simulink model "mode"  (R2021b)
settings: Solver=ode23s  StartTime=0.0  StopTime=50  RelTol=1e-3
model workspace (MAT data in the model file):
  firstWarning = 1
  originalScenarioChecksum = '114339432DE22364D47BB28FC96DC10C'
undefined symbols (not defined in the file or in its folder): Acceleration, ActorID, AngularVelocity, curvature, DefaultGear, DEND_B, DEND_S, DEND_T, direction, driving, gradbp, LF, LR, matlabshared, MAX_BRAKE, MAX_STEER, MAX_TORQUE, MCAR, MIN_BRAKE, MIN_STEER, MIN_TORQUE, NUMD_B, NUMD_S, NUMD_T, Pitch, point_intersection, Position, psi_o, R, Roll, RRdamp, scenario, sigbuilder_block, STEER_RATIO, stopSign_ID, Tdead, thetaRefs, TL_ID, TrackWidth, Ts, ts, Vdead, Velocity, X_o, xRef2s, Y_o, Yaw, yRef2s
libraries: drivingscenarioandsensors x4, drivingvehiclecontroller x2, simulink x2, simulink_extras x1, autolibshared x1, vehdynlibviscommon x1, vehdynlibsteering x1
(part 2 of 2)

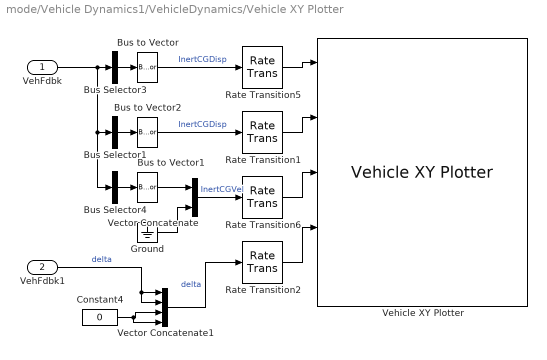
== system mode/Vehicle Dynamics1/VehicleDynamics/Vehicle XY Plotter ==
  VehFdbk : Inport
  VehFdbk1 : Inport  Port=2
  Bus Selector1 : BusSelector  OutputSignals=InertFrm.Cg.Ang.phi,InertFrm.Cg.Ang.theta,InertFrm.Cg.Ang.psi  OutputAsBus=on
  Bus Selector3 : BusSelector  OutputSignals=InertFrm.Geom.Disp.X,InertFrm.Geom.Disp.Y,InertFrm.Geom.Disp.Z  OutputAsBus=on
  Bus Selector4 : BusSelector  OutputSignals=InertFrm.Cg.Vel.Xdot,InertFrm.Cg.Vel.Ydot  OutputAsBus=on
  Bus to Vector : BusToVector
  Bus to Vector1 : BusToVector
  Bus to Vector2 : BusToVector
  Constant4 : Constant  Value=0
  Ground : Ground
  Rate Transition{1..2,5..6} (4 alike) : RateTransition  OutPortSampleTime=pltDT
  Vector Concatenate : Concatenate
  Vector Concatenate1 : Concatenate  NumInputs=4
  Vehicle XY Plotter : vehdynlibviscommon/Vehicle XY Plotter  w=w  a=a  b=b  figBorder=2000  bufferSize=bufferSize  extStats=off  extTireF=off
      settings: SourceProductName=The database C:\Users\jrodgers\AppData\Roaming\MathWorks\MATLAB\R2018b\slblocks_master.db is locked, or a table in the database is locked. (database is locked)
  wires:
  Bus to Vector2/1 -> Rate Transition1/1  "InertCGDisp"
  Rate Transition5/1 -> Vehicle XY Plotter/1
  Bus Selector4/1 -> Bus to Vector1/1
  Rate Transition1/1 -> Vehicle XY Plotter/2
  Rate Transition6/1 -> Vehicle XY Plotter/3
  Vector Concatenate/1 -> Rate Transition6/1  "InertCGVel"
  Bus Selector1/1 -> Bus to Vector2/1
  Bus to Vector/1 -> Rate Transition5/1  "InertCGDisp"
  Bus Selector3/1 -> Bus to Vector/1
  Bus to Vector1/1 -> Vector Concatenate/1
  Ground/1 -> Vector Concatenate/2
  VehFdbk/1 -> Bus Selector1/1, Bus Selector4/1, Bus Selector3/1
  Rate Transition2/1 -> Vehicle XY Plotter/4
  Constant4/1 -> Vector Concatenate1/4, Vector Concatenate1/3
  VehFdbk1/1 -> Vector Concatenate1/2, Vector Concatenate1/1  "delta"
  Vector Concatenate1/1 -> Rate Transition2/1  "delta"

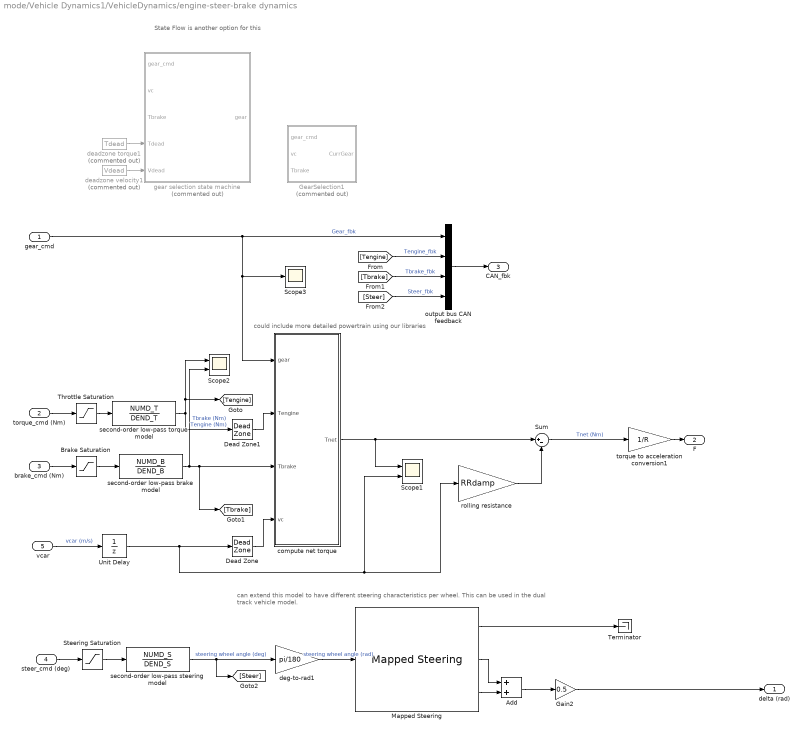
== system mode/Vehicle Dynamics1/VehicleDynamics/engine-steer-brake dynamics ==
  note: State Flow is another option for this
  note: could include more detailed powertrain using our libraries
  note: can extend this model to have different steering characteristics per wheel. This can be used in the dual track vehicle model.
  gear_cmd : Inport
  torque_cmd (Nm) : Inport  Port=2
  brake_cmd (Nm) : Inport  Port=3
  steer_cmd (deg) : Inport  Port=4
  vcar : Inport  Port=5
  Add : Sum
  Brake Saturation : Saturate  UpperLimit=MAX_BRAKE  LowerLimit=MIN_BRAKE
  Dead Zone : DeadZone  LowerValue=-Vdead  UpperValue=Vdead  SaturateOnIntegerOverflow=on
  Dead Zone1 : DeadZone  LowerValue=-Tdead  UpperValue=Tdead  SaturateOnIntegerOverflow=on
  Gain2 : Gain  Gain=0.5
  GearSelection1 : Stateflow chart  Commented=on  TreatAsAtomicUnit=on  SystemSampleTime=ts
      settings: PortSchema="{\"entries\":[{\"content\":{\"sides\":[{\"content\":{\"connectorIds\":[\"In3\",\"In2\",\"In1\"]},\"type\":\"ConnectorPlacement.EquallySpacedRectSide\",\"uuid\":\"465e5722-891f-481b-b3b6-2b8339e8e743\"},{\"content\":{\"connectorIds\":[\"Out1\"],\"side\":\"RIGHT\"},\"type\":\"ConnectorPlacement.EquallySpacedRectSide\",\"uuid\":\"28ef13cd-41d9-4e2e-8cd9-9157abf573a9\"},{\"content\":{\"connectorIds\":[],\"side\":\"TOP\"},\"type\":\"ConnectorPlacement.EquallySpacedRectSide\",\"uuid\":\"44f19923-60ae-466f-ad2a-756f1033b52e\"},{\"content\":{\"connectorIds\":[],\"side\":\"HIDDEN\"},\"type\":\"ConnectorPlacement.EquallySpacedRectSide\",\"uuid\":\"d5a146f0-4328-42be-94e3-09f51634e7da\"}]},\"type\":\"ConnectorPlacement.EquallySpacedConnector\",\"uuid\":\"14e271af-3da2-4f7d-9688-fcc3c9792006\"}],\"packageUris\":[\"http://schema.mathworks.com/mf0/Connector/R2020b\"],\"version\":\"1.0\"}"
  Mapped Steering : vehdynlibsteering/Mapped Steering  SpdDpd=off  StrgAngBpts=[-1.5*pi 1.5*pi]  WhlLftTbl=[-1.5*pi 1.5*pi]*STEER_RATIO  WhlRghtTbl=[-1.5*pi 1.5*pi]*STEER_RATIO  VehSpdBpts=[-1 1]  SpdFctTbl=[1 1]  aMode=2
      settings: SourceProductBaseCode=VE
  Scope1 : Scope  NumInputPorts=2
  Scope2 : Scope  NumInputPorts=2
  Scope3 : Scope
  Steering Saturation : Saturate  UpperLimit=MAX_STEER  LowerLimit=MIN_STEER
  Sum : Sum  Inputs=|+-
  Terminator : Terminator
  Throttle Saturation : Saturate  UpperLimit=MAX_TORQUE  LowerLimit=MIN_TORQUE
  Unit Delay : UnitDelay  SampleTime=-1  HasFrameUpgradeWarning=on
  compute net torque : MATLAB Function  TreatAsAtomicUnit=on  SystemSampleTime=ts
  deadzone torque1 : Constant  Commented=on  Value=Tdead  SampleTime=ts
  deadzone velocity1 : Constant  Commented=on  Value=Vdead  SampleTime=ts
  deg-to-rad1 : Gain  Gain=pi/180
  gear selection state machine : MATLAB Function  Commented=on  TreatAsAtomicUnit=on  SystemSampleTime=ts
  output bus CAN feedback : BusCreator  Inputs=4
  rolling resistance : Gain  Gain=RRdamp
  second-order low-pass brake model : DiscreteTransferFcn  Numerator=NUMD_B  Denominator=DEND_B  SampleTime=ts
  second-order low-pass steering model : DiscreteTransferFcn  Numerator=NUMD_S  Denominator=DEND_S  SampleTime=ts
  second-order low-pass torque model : DiscreteTransferFcn  Numerator=NUMD_T  Denominator=DEND_T  SampleTime=ts
  torque to acceleration conversion1 : Gain  Gain=1/R
  delta (rad) : Outport  VectorParamsAs1DForOutWhenUnconnected=off
  F : Outport  Port=2  VectorParamsAs1DForOutWhenUnconnected=off
  CAN_fbk : Outport  Port=3  VectorParamsAs1DForOutWhenUnconnected=off
  wires:
  steer_cmd (deg)/1 -> Steering Saturation/1
  torque_cmd (Nm)/1 -> Throttle Saturation/1
  brake_cmd (Nm)/1 -> Brake Saturation/1
  second-order low-pass steering model/1 -> deg-to-rad1/1, [Steer]  "steering wheel angle (deg)"
  Throttle Saturation/1 -> second-order low-pass torque model/1
  Brake Saturation/1 -> second-order low-pass brake model/1
  Steering Saturation/1 -> second-order low-pass steering model/1
  vcar/1 -> Unit Delay/1  "vcar (m/s)"
  second-order low-pass brake model/1 -> [Tbrake], compute net torque/3(Tbrake), Scope2/2  "Tbrake (Nm)"
  second-order low-pass torque model/1 -> Dead Zone1/1, [Tengine], Scope2/1  "Tengine (Nm)"
  compute net torque/1(Tnet) -> Scope1/1, Sum/1
  rolling resistance/1 -> Sum/2
  deadzone velocity1/1 -> gear selection state machine/5(Vdead)
  deadzone torque1/1 -> gear selection state machine/4(Tdead)
  gear_cmd/1 -> output bus CAN feedback/1, Scope3/1, compute net torque/1(gear)  "Gear_fbk"
  output bus CAN feedback/1 -> CAN_fbk/1
  [Tengine] -> output bus CAN feedback/2  "Tengine_fbk"
  [Tbrake] -> output bus CAN feedback/3  "Tbrake_fbk"
  [Steer] -> output bus CAN feedback/4  "Steer_fbk"
  Mapped Steering/2 -> Add/1
  Mapped Steering/3 -> Add/2
  Add/1 -> Gain2/1
  torque to acceleration conversion1/1 -> F/1
  Mapped Steering/1 -> Terminator/1
  deg-to-rad1/1 -> Mapped Steering/1  "steering wheel angle (rad)"
  Sum/1 -> torque to acceleration conversion1/1  "Tnet (Nm)"
  Dead Zone/1 -> compute net torque/4(vc)
  Dead Zone1/1 -> compute net torque/2(Tengine)
  Unit Delay/1 -> Scope1/2, rolling resistance/1, Dead Zone/1
  Gain2/1 -> delta (rad)/1

== stateflow chart mode/FSM ==
  state Set_Velocity
    entry:
    Velocity=10
  state Stop
    entry:
    Velocity=0
  (default) -> Set_Velocity
  Set_Velocity -> Stop : [distance==0]
  Stop -> Set_Velocity : after(3,sec)
  data: Velocity output; distance input

== matlab function mode/Vehicle Dynamics1/Info2ActorState/MATLAB Function ==
  data: X input; Position output; Y input; Z input
function Position = fcn(X, Y, Z)

Position = [X Y, Z];

== matlab function mode/MATLAB Function1 ==
  data: EVpos input; Scene output; SceneLocations input; Direction output; dist2scene input; dist output; angl output
function [Scene,Direction,dist,angl] = ScenarioFinder(EVpos,SceneLocations,dist2scene)

    % dist = zeros(1,length(SceneLocations));
    for j = 1:length(SceneLocations)
        distXY = SceneLocations(j,:) - EVpos(1:2);
        dist = norm(distXY);

        if (dist <= dist2scene)
            Scene = j;
            angl = atan2d(distXY(2),distXY(1));

            if angl < 0
                angl = angl + 360;
            end

            if (angl > 315) || (angl <= 45) 
                Direction = "N";
            elseif (angl > 225) && (angl <= 315)
                Direction = "E";
            elseif (angl > 135) && (angl <= 225)
                Direction = "S";
            elseif (angl > 45) && (angl <= 135)
                Direction = "W";
            else
                Direction = "Error";
            end
            break
        else
            Scene = 0;
            Direction = " ";
            angl = 1000;
        end

    end

== matlab function mode/Vehicle Dynamics1/Info2ActorState/MATLAB Function1 ==
  data: Xdot input; Velocity output; Ydot input; Zdot input
function Velocity = fcn(Xdot, Ydot, Zdot)

Velocity = [Xdot Ydot, Zdot];

== matlab function mode/Vehicle Dynamics1/Info2ActorState/MATLAB Function2 ==
  data: aX input; Acceleration output; aY input; aZ input
function Acceleration = fcn(aX, aY, aZ)

Acceleration = [aX aY, aZ];

== matlab function mode/Vehicle Dynamics1/Info2ActorState/MATLAB Function3 ==
  data: phiDot input; AngularVelocity output; thetaDot input; psiDot input
function AngularVelocity = fcn(phiDot, thetaDot, psiDot)

AngularVelocity = [phiDot thetaDot, psiDot];

== stateflow chart mode/Vehicle Dynamics1/VehicleDynamics/engine-steer-brake dynamics/GearSelection1 ==
  state Park
    CurrGear = 0;
  state Reverse
    CurrGear = -1;
  state drive
    CurrGear = 1;
  (default) -> (junction 12)
  (junction 12) -> Reverse [order 3] : [DefaultGear == -1]
  (junction 12) -> drive [order 2] : [DefaultGear == 1]
  (junction 12) -> Park [order 1] : [DefaultGear == 0]
  (junction 12) -> Park [order 4] : %fallback to park
  drive -> Park [order 2] : [gear_cmd == 0 && allowShift(vc,Tbrake)]
  Park -> Reverse [order 2] : [gear_cmd == -1 && allowShift(vc,Tbrake)]
  Park -> drive [order 1] : [gear_cmd == 1 && allowShift(vc,Tbrake)]
  Reverse -> Park [order 2] : [gear_cmd == 0 && allowShift(vc,Tbrake)]
  drive -> Reverse [order 1] : [gear_cmd == -1 && allowShift(vc,Tbrake)]
  Reverse -> drive [order 1] : [gear_cmd == 1 && allowShift(vc,Tbrake)]
  data: Tdead parameter; Vdead parameter; vel function_input; brakeT function_input; allow function_output; CurrGear output; Tbrake input; vc input; gear_cmd input; DefaultGear parameter
  function allow = allowShift(vel, brakeT):
    | function allow = allowShift(vel, brakeT)
    | allow = (abs(vel) <= Vdead) && (abs(brakeT)>Tdead);
    | end

== matlab function mode/Vehicle Dynamics1/VehicleDynamics/engine-steer-brake dynamics/compute net torque ==
  data: gear input; Tnet output; Tengine input; Tbrake input; vc input
function Tnet  = net_torque(gear,Tengine,Tbrake,vc)

%  --set engine torque based on current gear selection

if (gear == 0)
    %  --vehicle is in PARK, so force engine torque to zero
    Tengine = 0;
end

Tnet = Tengine + Tbrake*tanh(5*vc);

end

== matlab function mode/Vehicle Dynamics1/VehicleDynamics/engine-steer-brake dynamics/gear selection state machine ==
  data: gear output; gear_cmd input; vc input; Tbrake input; Tdead input; Vdead input
function gear = gear_change_FSM(gear_cmd,vc,Tbrake,Tdead,Vdead)

persistent GEAR

%  The vehicle gear can take on one of the following enumerated values:
%  -1 = REVERSE
%   0 = PARK
%   1 = DRIVE

%  --initialize the local persistent variables

if isempty(GEAR)
    %  --default gear at startup is PARK
    %  Note:  Change this to 1 if you want car to initialize in DRIVE
    GEAR = 0;
end


%  --evaluate the gear change finite state machine

switch GEAR
    case 0  % vehicle is in PARK
        if (gear_cmd == 1)
            %  --check to see if we can shift to DRIVE
            if ((abs(vc) <= Vdead) && (abs(Tbrake) > Tdead))
                %  --shift to DRIVE
                GEAR = 1;
            end
            
        elseif (gear_cmd == 2)
            %  --check to see if we can shift to REVERSE
            if ((abs(vc) <= Vdead) && (abs(Tbrake) > Tdead))
                %  --shift to REVERSE
                GEAR = 2;
            end
        end
        
    case 1  % vehicle is in DRIVE
        if (gear_cmd == 0)
            %  --check to see if we can shift to PARK
            if ((abs(vc) <= Vdead) && (abs(Tbrake) > Tdead))
                %  --shift to PARK
                GEAR = 0;
            end
            
        elseif (gear_cmd == 2)
            %  --check to see if we can shift to REVERSE
            if ((abs(vc) <= Vdead) && (abs(Tbrake) > Tdead))
                %  --shift to REVERSE
                GEAR = 2;
            end
        end
        
    case -1  % vehicle is in REVERSE
        if (gear_cmd == 0)
            %  --check to see if we can shift to PARK
            if ((abs(vc) <= Vdead) && (abs(Tbrake) > Tdead))
                %  --shift to PARK
                GEAR = 0;
            end
            
        elseif (gear_cmd == 1)
            %  --check to see if we can shift to DRIVE
            if ((abs(vc) <= Vdead) && (abs(Tbrake) > Tdead))
                %  --shift to DRIVE
                GEAR = 1;
            end
        end
        
    otherwise  %  --should never be here
        if (vc > Vdead)
            %  --moving forward, so must be in DRIVE
            GEAR = 1;
        elseif (vc < -Vdead)
            %  --moving backward, so must be in REVERSE
            GEAR = 2;
        else
            %  --vehicle stoppped, so must be in PARK
            GEAR = 0;
        end

end


%  --output the current actual gear setting

gear = GEAR;

return

== matlab function mode/Positions and States /MATLAB Function2 ==
  data: Actors input; ss_poses output; ss_State input

function ss_poses = findssposes(Actors, ss_State)

n=length(ss_State);
ss_poses=zeros(n,4);
indices=zeros(n,1);
ID=zeros(length(Actors),1);

for i=1:length(Actors)
 ID(i)=Actors(i).ActorID;
end

indices=find(ismember(ID,ss_State));
if(~isempty(indices))
    
    for i=1:n
        ss_poses(i,:)=([Actors(indices(i)).Position(:)',ss_State(i)]);
    end
end

ss_poses(ss_poses==0)=NaN;






% ss1_poses=zeros(1,4);
% ss2_poses=zeros(1,4);
% for i=1:length(Actors)
%     ID=Actors(i).ActorID;
%     
%     if(ID==ss1_State(1))
%         ss1_poses=[Actors(i).Position(:)',ss1_State(1)];
%     elseif ID== (ss1_State(2))
%         ss2_poses=[Actors(i).Position(:)',ss1_State(2)];
%     
%     end
%   
% end
% ss1_poses(ss1_poses==0)=NaN;   
% ss2_poses(ss2_poses==0)=NaN;

== matlab function mode/Positions and States /MATLAB Function1 ==
  data: Actors input; TL_poses output; TL_State input

function TL_poses = findTLposes(Actors, TL_State)
n=length(TL_State);
TL_poses=zeros(n/2,5);
indices=zeros(n/2,1);
ID=zeros(length(Actors),1);

for i=1:length(Actors)
 ID(i)=Actors(i).ActorID;
end

indices=find(ismember(ID,TL_State(n/2+1:end)));
if (~isempty(indices))

    for i=1:n/2
        TL_poses(i,:)=([Actors(indices(i)).Position(:)',TL_State(i),ID(indices(i))]);

    end
end
TL_poses(TL_poses==0)=NaN;

== stateflow chart mode/Positions and States /Traffic Light Sensor/Traffic Light Switching Logic ==
  state STEADYRED
    entry:
    trafficLight(:)= Red; TL_ID=TL_id;
  state STEADYGREEN
    entry:
    trafficLight(:)= Green; TL_ID=TL_id;
  state START
    entry:
    trafficLight=TL_id;
    trafficLight(:)= Black;TL_ID=TL_id;
  state TRAFFICLIGHT_ODDYELLOW_EVENRED
    entry:
    trafficLight(1:2:end)=Yellow;TL_ID(1:2:end)=TL_id(1:2:end);
    trafficLight(2:2:end) = Red;TL_ID(2:2:end)=TL_id(2:2:end);
  state TRAFFICLIGHT_ODDGREEN_EVENRED
    entry:
    trafficLight(1:2:end)=Green;TL_ID(1:2:end)=TL_id(1:2:end);
    trafficLight(2:2:end) = Red;TL_ID(2:2:end)=TL_id(2:2:end);
  state TRAFFICLIGHT_ODDRED_EVENYELLOW
    entry:
    trafficLight(1:2:end)=Red;TL_ID(1:2:end)=TL_id(1:2:end);
    trafficLight(2:2:end) = Yellow;TL_ID(2:2:end)=TL_id(2:2:end);
  state TRAFFICLIGHT_ODDRED_EVENGREEN
    entry:
    trafficLight(1:2:end)=Red;TL_ID(1:2:end)=TL_id(1:2:end);
    trafficLight(2:2:end) = Green;TL_ID(2:2:end)=TL_id(2:2:end);
  (default) -> START
  START -> STEADYGREEN [order 3] : [LightConfig==1]
  START -> STEADYRED [order 1] : [LightConfig==2]
  START -> TRAFFICLIGHT_ODDGREEN_EVENRED [order 2] : [LightConfig ==3]
  TRAFFICLIGHT_ODDGREEN_EVENRED -> TRAFFICLIGHT_ODDYELLOW_EVENRED : after(0.5,sec)
  TRAFFICLIGHT_ODDYELLOW_EVENRED -> TRAFFICLIGHT_ODDRED_EVENGREEN : after(0.5,sec)
  TRAFFICLIGHT_ODDRED_EVENYELLOW -> TRAFFICLIGHT_ODDGREEN_EVENRED : after(0.5,sec)
  TRAFFICLIGHT_ODDRED_EVENGREEN -> TRAFFICLIGHT_ODDRED_EVENYELLOW : after(0.5,sec)
  data: Green constant double =3; Red constant double =1; Yellow constant double =2; LightConfig input; TL_id input; Black constant double =0; TL_ID output; trafficLight output
